simulink model "Copy_of_attitude_observer_test"  (R2016b)
settings: Solver=VariableStepAuto  StartTime=0.0  StopTime=10.0  RelTol=1e-6
libraries: simulink x1
settings Model: Creator=liana  LastModifiedBy=liana

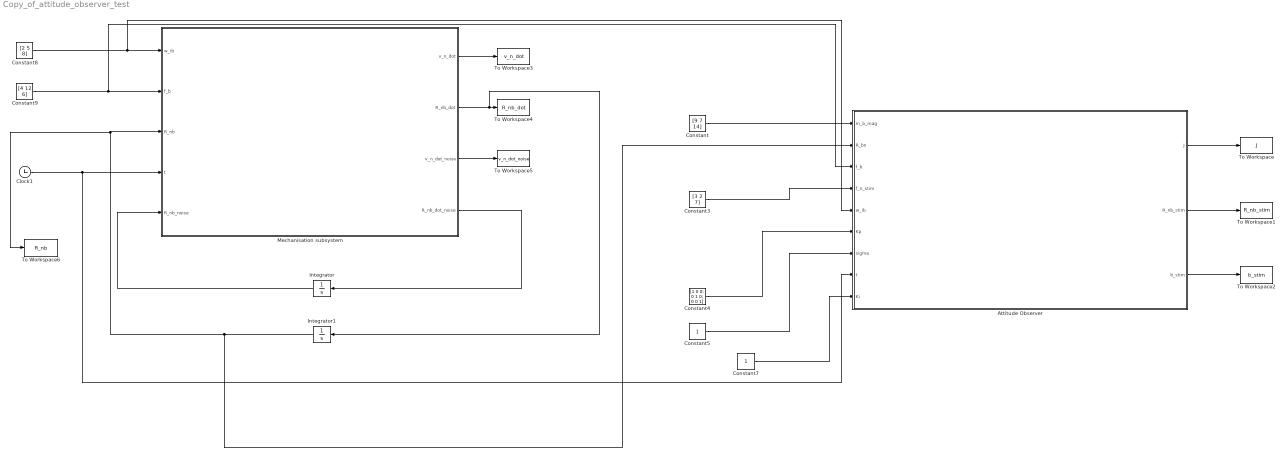
== system Copy_of_attitude_observer_test ==
  Attitude Observer : Subsystem
  Clock1 : Clock
  Constant : Constant  Value=[9 7 14]
  Constant3 : Constant  Value=[3 2 7]
  Constant4 : Constant  Value=[1 0 0; 0 1 0; 0 0 1]
  Constant5 : Constant
  Constant7 : Constant
  Constant8 : Constant  Value=[2 5 8]
  Constant9 : Constant  Value=[4 12 6]
  Integrator : Integrator
  Integrator1 : Integrator  InitialCondition=0.0000001
  Mechanisation subsystem : Subsystem
  To Workspace : ToWorkspace  VariableName=J  SampleTime=-1
  To Workspace1 : ToWorkspace  VariableName=R_nb_stim  SampleTime=-1
  To Workspace2 : ToWorkspace  VariableName=b_stim  SampleTime=-1
  To Workspace3 : ToWorkspace  VariableName=v_n_dot  SampleTime=-1
  To Workspace4 : ToWorkspace  VariableName=R_nb_dot  SampleTime=-1
  To Workspace5 : ToWorkspace  VariableName=v_n_dot_noise  SampleTime=-1
  To Workspace6 : ToWorkspace  VariableName=R_nb  SampleTime=-1
  wires:
  Constant/1 -> Attitude Observer/1(m_b_mag)
  Integrator1/1 -> Attitude Observer/2(R_bn), To Workspace6/1, Mechanisation subsystem/3(R_nb)
  Constant9/1 -> Attitude Observer/3(f_b), Mechanisation subsystem/2(f_b)
  Constant3/1 -> Attitude Observer/4(f_n_stim)
  Constant4/1 -> Attitude Observer/6(Kp)
  Constant5/1 -> Attitude Observer/7(sigma)
  Constant8/1 -> Attitude Observer/5(w_ib), Mechanisation subsystem/1(w_ib)
  Constant7/1 -> Attitude Observer/9(Ki)
  Clock1/1 -> Attitude Observer/8(t), Mechanisation subsystem/4(t)
  Attitude Observer/1(J) -> To Workspace/1
  Attitude Observer/2(R_nb_stim) -> To Workspace1/1
  Attitude Observer/3(b_stim) -> To Workspace2/1
  Mechanisation subsystem/2(R_nb_dot) -> Integrator1/1, To Workspace4/1
  Mechanisation subsystem/4(R_nb_dot_noise) -> Integrator/1
  Integrator/1 -> Mechanisation subsystem/5(R_nb_noise)
  Mechanisation subsystem/1(v_n_dot) -> To Workspace3/1
  Mechanisation subsystem/3(v_n_dot_noise) -> To Workspace5/1

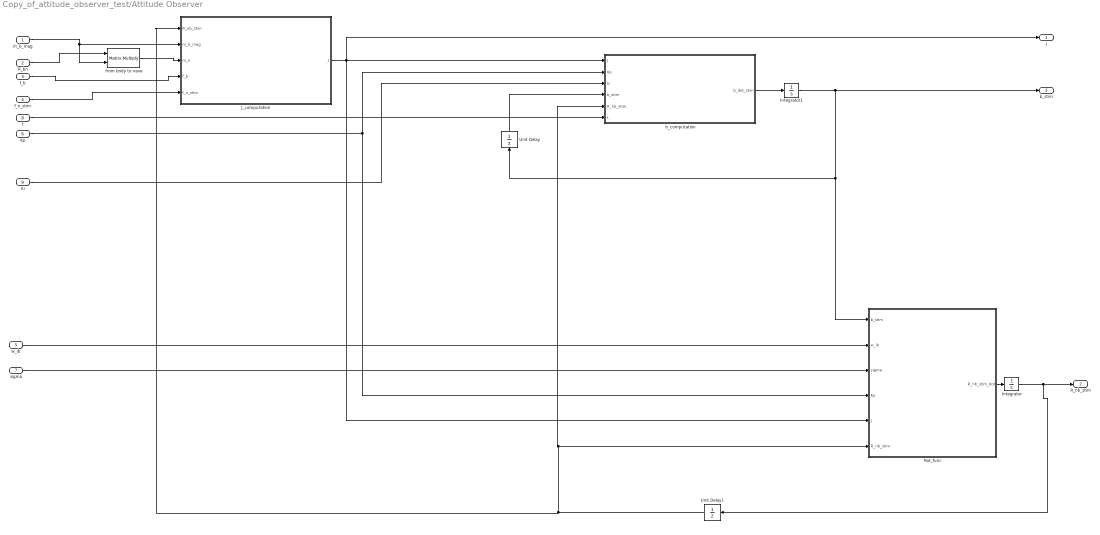
== system Copy_of_attitude_observer_test/Attitude Observer ==
  m_b_mag : Inport
  R_bn : Inport  Port=2
  f_b : Inport  Port=3
  f_n_stim : Inport  Port=4
  w_ib : Inport  Port=5
  Kp : Inport  Port=6
  sigma : Inport  Port=7
  t : Inport  Port=8
  Ki : Inport  Port=9
  Integrator : Integrator  InitialCondition=0.000001
  Integrator1 : Integrator
  J_computation : Subsystem
  Rot_func : MATLAB Function  TreatAsAtomicUnit=on
  Unit Delay : UnitDelay  SampleTime=-1
  Unit Delay1 : UnitDelay  SampleTime=-1
  b_computation : MATLAB Function  TreatAsAtomicUnit=on
  from body to nave : Product  Multiplication=Matrix(*)
  J : Outport
  R_nb_stim : Outport  Port=2
  b_stim : Outport  Port=3
  wires:
  m_b_mag/1 -> from body to nave/2, J_computation/2(m_b_mag)
  Rot_func/1(R_nb_stim_dot) -> Integrator/1
  b_computation/1(b_dot_stim) -> Integrator1/1
  Integrator1/1 -> Unit Delay/1, Rot_func/1(b_stim), b_stim/1
  from body to nave/1 -> J_computation/3(m_n)
  f_b/1 -> J_computation/4(f_b)
  f_n_stim/1 -> J_computation/5(f_n_stim)
  J_computation/1(J) -> J/1, Rot_func/5(J), b_computation/1(J)
  Kp/1 -> Rot_func/4(Kp), b_computation/2(Kp)
  Ki/1 -> b_computation/3(ki)
  sigma/1 -> Rot_func/3(sigma)
  w_ib/1 -> Rot_func/2(w_ib)
  R_bn/1 -> from body to nave/1
  t/1 -> b_computation/6(t)
  Integrator/1 -> R_nb_stim/1, Unit Delay1/1
  Unit Delay/1 -> b_computation/4(b_stim)
  Unit Delay1/1 -> J_computation/1(R_nb_stim), b_computation/5(R_nb_stim), Rot_func/6(R_nb_stim)

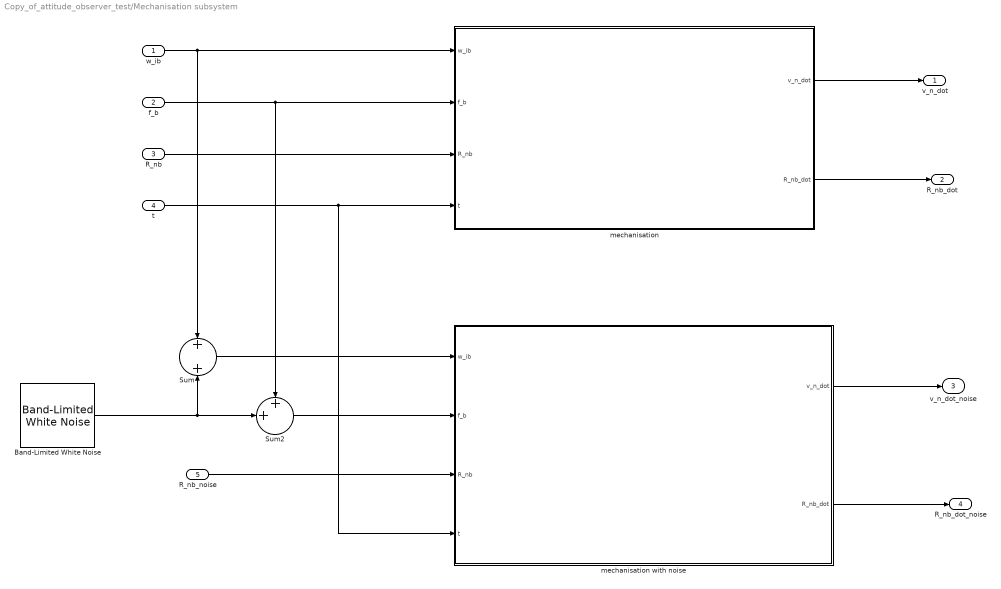
== system Copy_of_attitude_observer_test/Mechanisation subsystem ==
  w_ib : Inport
  f_b : Inport  Port=2
  R_nb : Inport  Port=3
  t : Inport  Port=4
  R_nb_noise : Inport  Port=5
  Band-Limited White Noise : simulink/Sources/Band-Limited White Noise  Cov=[100 100 100]'  Ts=0.1  seed=[23341]  VectorParams1D=off
  Sum : Sum  Inputs=+|+
  Sum2 : Sum  Inputs=++|
  mechanisation : MATLAB Function  TreatAsAtomicUnit=on
  mechanisation with noise : MATLAB Function  TreatAsAtomicUnit=on
  v_n_dot : Outport
  R_nb_dot : Outport  Port=2
  v_n_dot_noise : Outport  Port=3
  R_nb_dot_noise : Outport  Port=4
  wires:
  w_ib/1 -> mechanisation/1(w_ib), Sum/1
  t/1 -> mechanisation with noise/4(t), mechanisation/4(t)
  R_nb/1 -> mechanisation/3(R_nb)
  f_b/1 -> Sum2/1, mechanisation/2(f_b)
  mechanisation/1(v_n_dot) -> v_n_dot/1
  mechanisation/2(R_nb_dot) -> R_nb_dot/1
  Band-Limited White Noise/1 -> Sum/2, Sum2/2
  Sum/1 -> mechanisation with noise/1(w_ib)
  Sum2/1 -> mechanisation with noise/2(f_b)
  mechanisation with noise/1(v_n_dot) -> v_n_dot_noise/1
  mechanisation with noise/2(R_nb_dot) -> R_nb_dot_noise/1
  R_nb_noise/1 -> mechanisation with noise/3(R_nb)

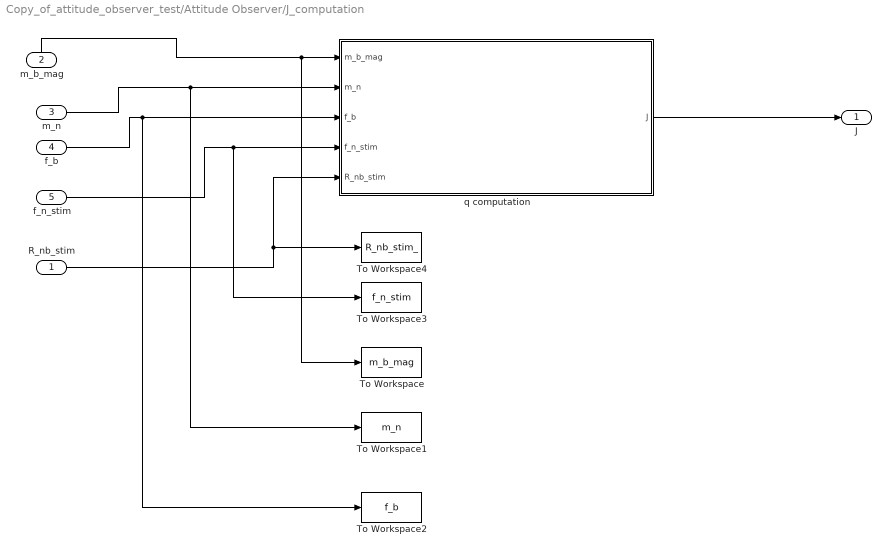
== system Copy_of_attitude_observer_test/Attitude Observer/J_computation ==
  R_nb_stim : Inport
  m_b_mag : Inport  Port=2
  m_n : Inport  Port=3
  f_b : Inport  Port=4
  f_n_stim : Inport  Port=5
  To Workspace : ToWorkspace  VariableName=m_b_mag  SampleTime=-1
  To Workspace1 : ToWorkspace  VariableName=m_n  SampleTime=-1
  To Workspace2 : ToWorkspace  VariableName=f_b  SampleTime=-1
  To Workspace3 : ToWorkspace  VariableName=f_n_stim  SampleTime=-1
  To Workspace4 : ToWorkspace  VariableName=R_nb_stim_  SampleTime=-1
  q computation : MATLAB Function  TreatAsAtomicUnit=on
  J : Outport
  wires:
  m_n/1 -> q computation/2(m_n), To Workspace1/1
  f_n_stim/1 -> To Workspace3/1, q computation/4(f_n_stim)
  m_b_mag/1 -> To Workspace/1, q computation/1(m_b_mag)
  f_b/1 -> To Workspace2/1, q computation/3(f_b)
  q computation/1(J) -> J/1
  R_nb_stim/1 -> q computation/5(R_nb_stim), To Workspace4/1

== matlab function Copy_of_attitude_observer_test/Attitude Observer/J_computation/q computation ==
  data: m_b_mag input; m_n input; f_b input; f_n_stim input size=3; J output; R_nb_stim input size=[3,3]
function J  = qEfunc(m_b_mag, m_n, f_b, f_n_stim, R_nb_stim)

g_n = [0 0 9.81]';

q1_b = m_b_mag/norm(m_b_mag,2);
q2_b = f_b/norm(g_n,2);

q1_n = m_n/norm(m_n,2);
q2_n = f_n_stim/norm(g_n,2);


E_b = [q1_b, skew(q1_b)*q2_b, (skew(q1_b)*skew(q1_b))*q2_b];
E_n = [q1_n, skew(q1_n)*q2_n, (skew(q1_n)*skew(q1_n))*q2_n];

J = (E_n - R_nb_stim * E_b) * (E_b');

end

== matlab function Copy_of_attitude_observer_test/Mechanisation subsystem/mechanisation ==
  data: w_ib input; f_b input; v_n_dot output; R_nb_dot output; R_nb input; t input
function [v_n_dot, R_nb_dot] = mechanisation(w_ib, f_b, R_nb, t)



g_n = [0 0 9.81]';

% w_ib = size(3,1);

if t == 0
    v_n_dot = ones(3,1);
    R_nb_dot = eye(3);
    R_nb = eye(3);
end

% mechanisation

% Skew = zeros(3,3);
% Skew(1,2) = -w_ib(3);
% Skew(2,1) = w_ib(3);
% Skew(1,3) = w_ib(2);
% Skew(3,1) = -w_ib(2);
% Skew(2,3) = -w_ib(1);
% Skew(3,2) = w_ib(1);

Skew = skew(w_ib);


%p_dot = v_n;
v_n_dot = R_nb * f_b + g_n;
R_nb_dot = R_nb * Skew;

end

== matlab function Copy_of_attitude_observer_test/Mechanisation subsystem/mechanisation with noise ==
  data: w_ib input; f_b input; v_n_dot output; R_nb_dot output; R_nb input; t input
function [v_n_dot, R_nb_dot] = mechanisation(w_ib, f_b, R_nb, t)



g_n = [0 0 1]';

% w_ib = size(3,1);

if t == 0
    v_n_dot = zeros(3,1);
    R_nb_dot = eye(3);
    R_nb = eye(3);
end

% mechanisation

% Skew = zeros(3,3);
% Skew(1,2) = -w_ib(3);
% Skew(2,1) = w_ib(3);
% Skew(1,3) = w_ib(2);
% Skew(3,1) = -w_ib(2);
% Skew(2,3) = -w_ib(1);
% Skew(3,2) = w_ib(1);
Skew = skew(w_ib);


%p_dot = v_n;
v_n_dot = R_nb * f_b + g_n;
R_nb_dot = R_nb * Skew;

== matlab function Copy_of_attitude_observer_test/Attitude Observer/b_computation ==
  data: J input; b_dot_stim output size=3; Kp input; ki input; b_stim input; R_nb_stim input; t input
function b_dot_stim = b_dot_stim_func(J, Kp, ki, b_stim, R_nb_stim, t)

% don't break balls if there are too rows

%b_dot_stim = zeros(3 ,1);

if t == 0
   
    b_stim = zeros(3, 1);
    
end

SAT = sat(R_nb_stim)';
PA = pa( SAT * Kp * J);
VEX = vexfunc(PA);
b_dot_stim = Proj(b_stim , (-ki * VEX));

end

== matlab function Copy_of_attitude_observer_test/Attitude Observer/Rot_func ==
  data: b_stim input; R_nb_stim_dot output; w_ib input; sigma input; Kp input; J input; R_nb_stim input
function R_nb_stim_dot = rot_func(b_stim,w_ib,sigma,Kp,J,R_nb_stim) 

Skew = skew(w_ib - b_stim);

R_nb_stim_dot = R_nb_stim * Skew + sigma * Kp * J;

end
